simulink subsystem "Send_GCS_Data"  (R2025a)
settings: Solver=VariableStepAuto  StartTime=0.0  StopTime=10.0  RelTol=1e-3
libraries: px4uORBlib x2
settings Model: Creator=gurt1  LastModifiedBy=17036

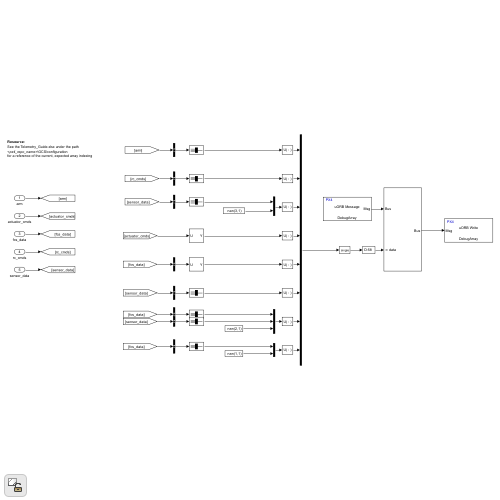
[thumbnail: Simulink's stored preview of the top-level diagram]
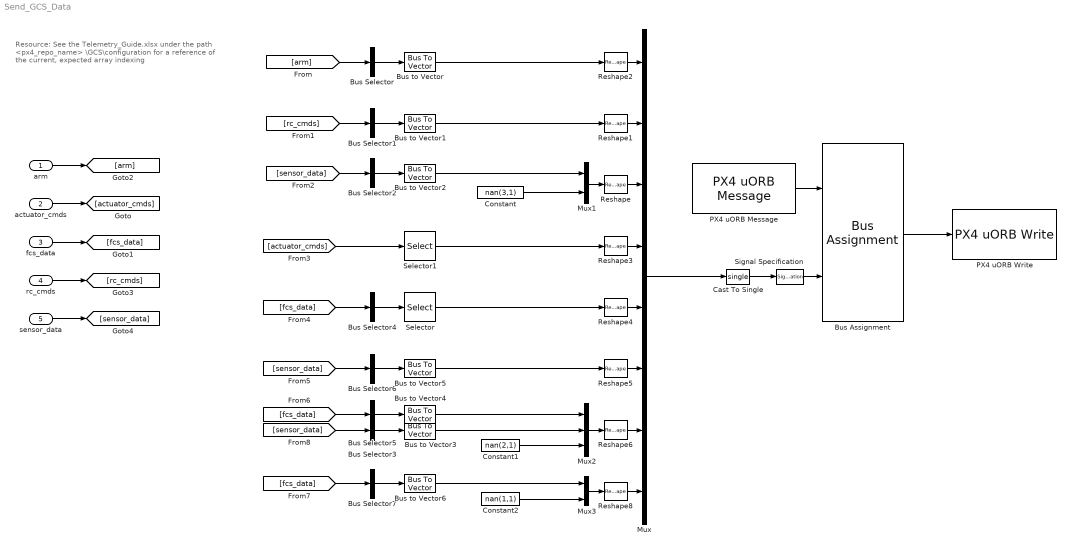
== system Send_GCS_Data ==
  note: Resource:
      | See the Telemetry_Guide.xlsx under the path
      | <px4_repo_name> \GCS\configuration
      | for a reference of the current, expected array indexing
  arm : Inport
  actuator_cmds : Inport  Port=2
  fcs_data : Inport  Port=3
  rc_cmds : Inport  Port=4
  sensor_data : Inport  Port=5
  Bus Assignment : BusAssignment  AssignedSignals=data
  Bus Selector : BusSelector  OutputSignals=dt_arm  OutputAsBus=on
  Bus Selector1 : BusSelector  OutputSignals=sticks.R_stick_lat,sticks.R_stick_lon,sticks.L_stick_lat,sticks.L_stick_lon,switches.D2,switches.E,switches.B,switches.G,switches.F,switches.H,switches.R_knob,switches.A  OutputAsBus=on
  Bus Selector2 : BusSelector  OutputSignals=alt_m,vt_kts,rho_kgmp3,flags.GC,flags.LiDAR_online  OutputAsBus=on
  Bus Selector3 : BusSelector  OutputSignals=esc.1.error_count,esc.2.error_count,esc.3.error_count,esc.4.error_count  OutputAsBus=on
  Bus Selector4 : BusSelector  OutputSignals=eng_cmds  OutputAsBus=on
  Bus Selector5 : BusSelector  OutputSignals=exp_ctrl_data.OL_cmds.att_rad.x,exp_ctrl_data.OL_cmds.att_rad.y,exp_ctrl_data.OL_cmds.ang_rps.z,exp_ctrl_data.OL_cmds.thrust_N,exp_ctrl_data.IL_cmds.torque_Nm.x,exp_ctrl_data.IL_cmds.torque_Nm.y,exp_ctrl_data.IL_cmds.torque_Nm.z  OutputAsBus=on
  Bus Selector6 : BusSelector  OutputSignals=esc.1.rpm,esc.2.rpm,esc.3.rpm,esc.4.rpm,esc.1.current,esc.2.current,esc.3.current,esc.4.current  OutputAsBus=on
  Bus Selector7 : BusSelector  OutputSignals=OL_PTI.t_gcs,OL_PTI.pti_doub_amp,OL_PTI.pti_doub_t,OL_PTI.pti_ms_amp,OL_PTI.pti_ms_t,OL_PTI.pti_swp_amp,OL_PTI.pti_swp_t  OutputAsBus=on
  Bus to Vector{,1..6} (7 alike) : BusToVector
  Cast To Single : DataTypeConversion  OutDataTypeStr=single  SaturateOnIntegerOverflow=off  RndMeth=Floor
  Constant : Constant  Value=nan(3,1)
  Constant1 : Constant  Value=nan(2,1)
  Constant2 : Constant  Value=nan(1,1)
  Mux : Mux  Inputs=8
  Mux1 : Mux  Inputs=2
  Mux2 : Mux  Inputs=3
  Mux3 : Mux  Inputs=2
  PX4 uORB Message : px4uORBlib/PX4 uORB Message  uORBTopic=DebugArray  SampleTime=-1  selectInstance=DebugArray
  PX4 uORB Write : px4uORBlib/PX4 uORB Write  uORBTopic=DebugArray  selectInstance=DebugArray  MessageQueueLen=1
  Reshape{,1..6,8} (8 alike) : Reshape
  Selector : Selector  InputPortWidth=16  IndexOptions=Index vector (dialog)  Indices=[1:4]  OutputSizes=1
  Selector1 : Selector  InputPortWidth=16  IndexOptions=Index vector (dialog)  Indices=[1:4]  OutputSizes=1
  Signal Specification : SignalSpecification  Dimensions=58
  wires:
  actuator_cmds/1 -> [actuator_cmds]
  arm/1 -> [arm]
  fcs_data/1 -> [fcs_data]
  sensor_data/1 -> [sensor_data]
  rc_cmds/1 -> [rc_cmds]
  PX4 uORB Message/1 -> Bus Assignment/1
  Cast To Single/1 -> Signal Specification/1
  Mux/1 -> Cast To Single/1
  Bus Assignment/1 -> PX4 uORB Write/1
  [arm] -> Bus Selector/1
  Bus Selector/1 -> Bus to Vector/1
  Bus to Vector/1 -> Reshape2/1
  [rc_cmds] -> Bus Selector1/1
  Bus Selector1/1 -> Bus to Vector1/1
  Bus to Vector1/1 -> Reshape1/1
  [sensor_data] -> Bus Selector2/1
  Bus Selector2/1 -> Bus to Vector2/1
  Mux1/1 -> Reshape/1
  Bus to Vector2/1 -> Mux1/1
  Constant/1 -> Mux1/2
  Selector1/1 -> Reshape3/1
  Selector/1 -> Reshape4/1
  [fcs_data] -> Bus Selector5/1
  Bus Selector5/1 -> Bus to Vector4/1
  Bus to Vector4/1 -> Mux2/1
  Bus to Vector3/1 -> Mux2/2
  Mux2/1 -> Reshape6/1
  Signal Specification/1 -> Bus Assignment/2
  [sensor_data] -> Bus Selector6/1
  Bus Selector6/1 -> Bus to Vector5/1
  Bus to Vector5/1 -> Reshape5/1
  Reshape/1 -> Mux/3
  Reshape1/1 -> Mux/2
  Reshape2/1 -> Mux/1
  Reshape3/1 -> Mux/4
  Reshape4/1 -> Mux/5
  Reshape5/1 -> Mux/6
  Reshape6/1 -> Mux/7
  [fcs_data] -> Bus Selector7/1
  Mux3/1 -> Reshape8/1
  Bus Selector7/1 -> Bus to Vector6/1
  Constant2/1 -> Mux3/2
  Bus to Vector6/1 -> Mux3/1
  Reshape8/1 -> Mux/8
  [fcs_data] -> Bus Selector4/1
  Bus Selector4/1 -> Selector/1
  [actuator_cmds] -> Selector1/1
  [sensor_data] -> Bus Selector3/1
  Bus Selector3/1 -> Bus to Vector3/1
  Constant1/1 -> Mux2/3
